simulink model "PreLab_4_sim"  (R2023b)
settings: Solver=ode45  StartTime=0.0  StopTime=tf  MaxStep=maxstep  RelTol=tol  AbsTol=tol
values from neighbouring files (symbols this model uses):
  a1 = 2    [Prelab_4.m]    (also in main.m = 3.25)
  A1 = 30    [Prelab_4.m]    (also in main.m = 0.110446616728)
  a2 = 2    [Prelab_4.m]    (also in main.m = 3.25)
  A2 = 30    [Prelab_4.m]    (also in main.m = 0.0490873852123)
  Aout1 = (pi/4)*(0.25^2)    (= 0.0490873852123)    [Prelab_4.m]    (also in main.m)
  Aout2 = (pi/4)*(0.125^2)    (= 0.0122718463031)    [Prelab_4.m]    (also in main.m)
  b1 = 0.5    [Prelab_4.m]    (also in main.m)
  b2 = 0.5    [Prelab_4.m]    (also in main.m; tankDataLower.mat = 1.41138888889)
  Cd1 = 0.7    [Prelab_4.m]    (also in main.m = Cd_upper)
  Cd2 = 0.9    [Prelab_4.m]    (also in main.m = Cd_lower)
  g = g*12    (= 386.4)    [Prelab_4.m]    (also in lab4_perf_index_lower.m; main.m; tankmodel_lower.m; tankmodel_upper.m)
  h10 = 7    [Prelab_4.m]    (also in main.m)
  h20 = 3    [Prelab_4.m]    (also in main.m)
settings Model: Creator=cotellkp  LastModifiedBy=kevin
settings SolverCC: AutoScaleAbsTol=off
settings DataIOCC: SaveOutput=off  SignalLogging=off  DSMLogging=off  SaveTime=off  ReturnWorkspaceOutputs=off

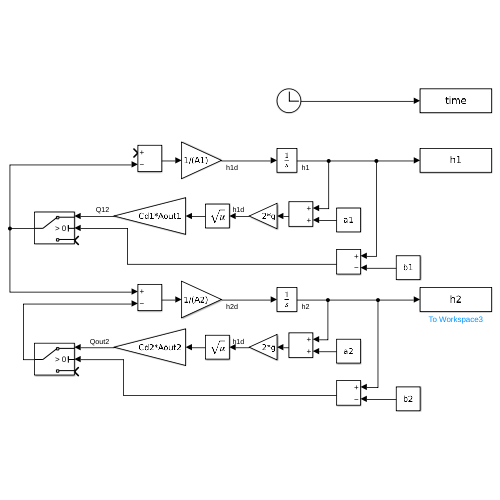
[thumbnail: Simulink's stored preview of the top-level diagram]
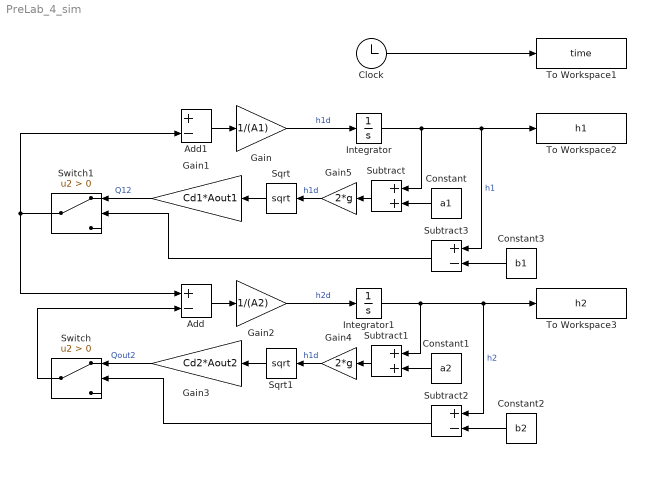
== system PreLab_4_sim ==
  Add : Sum  Inputs=+-
  Add1 : Sum  Inputs=+-
  Clock : Clock
  Constant : Constant  Value=a1
  Constant1 : Constant  Value=a2
  Constant2 : Constant  Value=b2
  Constant3 : Constant  Value=b1
  Gain : Gain  Gain=1/(A1)
  Gain1 : Gain  Gain=Cd1*Aout1
  Gain2 : Gain  Gain=1/(A2)
  Gain3 : Gain  Gain=Cd2*Aout2
  Gain4 : Gain  Gain=2*g
  Gain5 : Gain  Gain=2*g
  Integrator : Integrator  InitialCondition=h10
  Integrator1 : Integrator  InitialCondition=h20
  Sqrt : Sqrt
  Sqrt1 : Sqrt
  Subtract : Sum
  Subtract1 : Sum
  Subtract2 : Sum  Inputs=+-
  Subtract3 : Sum  Inputs=+-
  Switch : Switch  Criteria=u2 > Threshold  SaturateOnIntegerOverflow=off  InputSameDT=off
  Switch1 : Switch  Criteria=u2 > Threshold  SaturateOnIntegerOverflow=off  InputSameDT=off
  To Workspace1 : ToWorkspace  VariableName=time  SampleTime=-1
      settings: Save2DSignal=2-D array (concatenate along first dimension)
  To Workspace2 : ToWorkspace  VariableName=h1  SampleTime=-1
      settings: Save2DSignal=2-D array (concatenate along first dimension)
  To Workspace3 : ToWorkspace  VariableName=h2  SampleTime=-1
      settings: Save2DSignal=2-D array (concatenate along first dimension)
  wires:
  Clock/1 -> To Workspace1/1
  Gain/1 -> Integrator/1  "h1d"
  Integrator/1 -> Subtract3/1, To Workspace2/1, Subtract/1  "h1"
  Sqrt/1 -> Gain1/1
  Sqrt1/1 -> Gain3/1
  Integrator1/1 -> To Workspace3/1, Subtract2/1, Subtract1/1  "h2"
  Gain2/1 -> Integrator1/1  "h2d"
  Add/1 -> Gain2/1
  Add1/1 -> Gain/1
  Gain5/1 -> Sqrt/1  "h1d"
  Subtract/1 -> Gain5/1
  Gain4/1 -> Sqrt1/1  "h1d"
  Subtract1/1 -> Gain4/1
  Constant1/1 -> Subtract1/2
  Constant/1 -> Subtract/2
  Switch/1 -> Add/2
  Gain3/1 -> Switch/1  "Qout2"
  Constant2/1 -> Subtract2/2
  Subtract2/1 -> Switch/2
  Switch1/1 -> Add/1, Add1/2
  Gain1/1 -> Switch1/1  "Q12"
  Constant3/1 -> Subtract3/2
  Subtract3/1 -> Switch1/2
